simulink model "Assignment4p1"  (R2022a)
settings: Solver=VariableStepAuto  StartTime=0.0  StopTime=25  RelTol=1e-3
undefined symbols (not defined in the file or in its folder): m, n
settings Model: Creator=Philip  LastModifiedBy=Philip

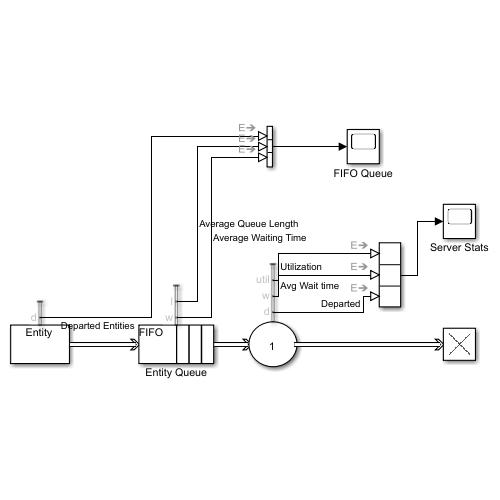
[thumbnail: Simulink's stored preview of the top-level diagram]
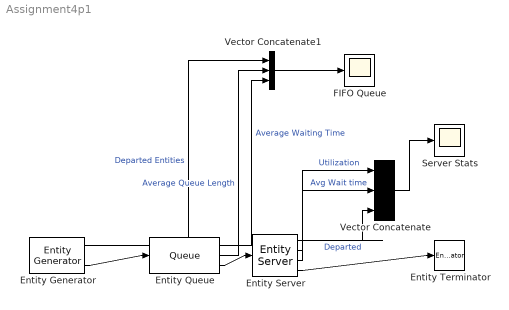
== system Assignment4p1 ==
  Entity Generator : EntityGenerator  OutputPortMessageModes=n,m  NumberEntitiesDeparted=on  EntityType=Structured  EntityTypeName=Entity
      settings: OutputPortMap=o0,o3
  Entity Queue : Queue  InputPortMessageModes=m  OutputPortMessageModes=n,n,m  Capacity=Inf  AverageWait=on  AverageQueueLength=on
      settings: OutputPortMap=o2,o3,o5
  Entity Server : EntityServer  InputPortMessageModes=m  OutputPortMessageModes=n,n,n,m  Capacity=1  NumberEntitiesDeparted=on  AverageWait=on  Utilization=on
      settings: OutputPortMap=o0,o4,o5,o9
  Entity Terminator : EntityTerminator  InputPortMessageModes=m
  FIFO Queue : Scope
  Server Stats : Scope
  Vector Concatenate : Concatenate  NumInputs=3
  Vector Concatenate1 : Concatenate  NumInputs=3
  wires:
  Entity Queue/3 -> Entity Server/1
  Entity Server/4 -> Entity Terminator/1
  Entity Generator/2 -> Entity Queue/1
  Entity Server/3 -> Vector Concatenate/1  "Utilization"
  Entity Server/1 -> Vector Concatenate/3  "Departed"
  Vector Concatenate/1 -> Server Stats/1
  Entity Server/2 -> Vector Concatenate/2  "Avg Wait time"
  Entity Generator/1 -> Vector Concatenate1/1  "Departed Entities"
  Entity Queue/2 -> Vector Concatenate1/2  "Average Queue Length"
  Entity Queue/1 -> Vector Concatenate1/3  "Average Waiting Time"
  Vector Concatenate1/1 -> FIFO Queue/1
